simulink model "lab2Sim"  (R2024b)
settings: Solver=VariableStepAuto  StartTime=0.0  StopTime=10.0  MaxStep=5  RelTol=1e-3
values from neighbouring files (symbols this model uses):
  cpp = 1000    [ident.m]    (also in lab2.m)
  Cvs = (cps * ros * Vs)    (= 9240000)    [ident.m]    (also in lab2.m = 92400)
  Cvw = (cpp * rop * Vw)    (= 150000)    [ident.m]    (also in lab2.m)
  czas_skok = 20000    [ident.m]    (also in lab2.m = 10000)
  dFp = 0    [ident.m]    (also in lab2.m)
  dPg = 0.1 * Pg0    (= 800)    [ident.m]    (also in lab2.m = 0)
  dTzew = 0    [ident.m]    (also in lab2.m = 1)
  Fp0 = FpN * 1.0    (= 0.0694444444444)    [ident.m]    (also in lab2.m = 0)
  Ks = Px/(TsN - TzewN)    (= 133.333333333)    [ident.m]    (also in lab2.m)
  Kw = Px/(TwewN - TsN)    (= 933.333333333)    [ident.m]    (also in lab2.m)
  Pg0 = PgN * 1.0    (= 8000)    [ident.m]    (also in lab2.m)
  rop = 1.2    [ident.m]    (also in lab2.m)
  Ts0 = (Kw*Twew0 + Ks*Tzew0) / (Kw + Ks)    (= 15)    [ident.m]    (also in lab2.m = 40)
  Twew0 = (Pg0 + Tzew0*(cpp*rop*Fp0 + ((Ks*Kw)/(Kw + Ks)))) / (cpp*rop*Fp0 + ((Kw * Ks)/(Kw + Ks)))    (= 20)    [ident.m]    (also in lab2.m = 48.5714285714)
  Tzew0 = TzewN    (= -20)    [ident.m]    (also in lab2.m)
settings Model: Creator=Michal  LastModifiedBy=Michal
settings DataIOCC: ReturnWorkspaceOutputs=off

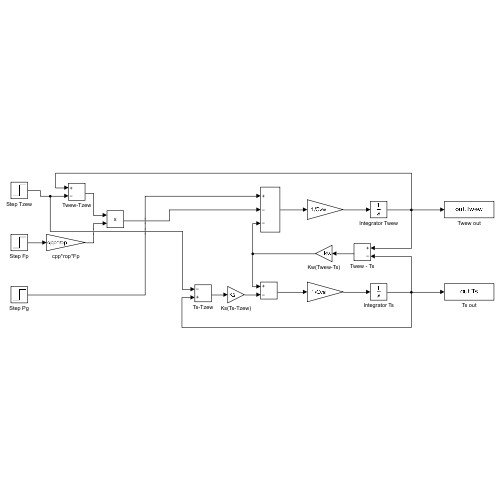
[thumbnail: Simulink's stored preview of the top-level diagram]
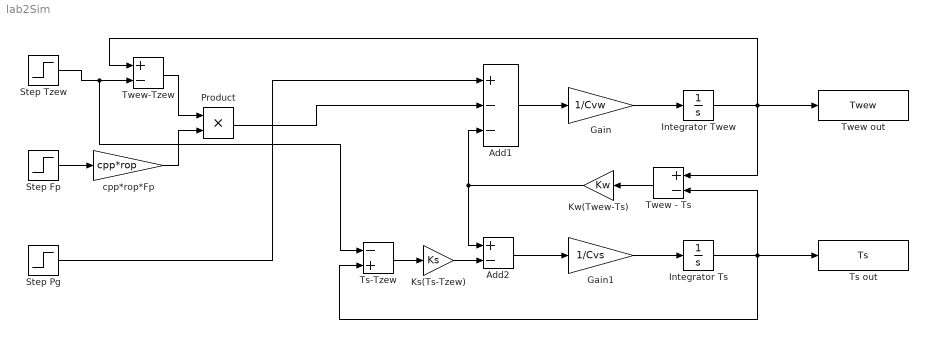
== system lab2Sim ==
  Add1 : Sum  Inputs=+--
  Add2 : Sum  Inputs=+-
  Gain : Gain  Gain=1/Cvw
  Gain1 : Gain  Gain=1/Cvs
  Integrator Ts : Integrator  InitialCondition=Ts0
  Integrator Twew : Integrator  InitialCondition=Twew0
  Ks(Ts-Tzew) : Gain  Gain=Ks
  Kw(Twew-Ts) : Gain  Gain=Kw
  Product : Product
  Step Fp : Step  Time=czas_skok  Before=Fp0  After=Fp0+dFp  SampleTime=0
  Step Pg : Step  Time=czas_skok  Before=Pg0  After=Pg0+dPg  SampleTime=0
  Step Tzew : Step  Time=czas_skok  Before=Tzew0  After=Tzew0+dTzew  SampleTime=0
  Ts out : ToWorkspace  VariableName=Ts  SampleTime=-1
  Ts-Tzew : Sum  Inputs=-+
  Twew - Ts : Sum  Inputs=+-
  Twew out : ToWorkspace  VariableName=Twew  SampleTime=-1
  Twew-Tzew : Sum  Inputs=+-
  cpp*rop*Fp : Gain  Gain=cpp*rop
  wires:
  Integrator Twew/1 -> Twew out/1, Twew-Tzew/1, Twew - Ts/1
  Integrator Ts/1 -> Ts out/1, Twew - Ts/2, Ts-Tzew/2
  Gain/1 -> Integrator Twew/1
  Gain1/1 -> Integrator Ts/1
  Add1/1 -> Gain/1
  Add2/1 -> Gain1/1
  Twew - Ts/1 -> Kw(Twew-Ts)/1
  Step Pg/1 -> Add1/1
  Kw(Twew-Ts)/1 -> Add2/1, Add1/3
  Step Tzew/1 -> Ts-Tzew/1, Twew-Tzew/2
  Step Fp/1 -> cpp*rop*Fp/1
  Twew-Tzew/1 -> Product/1
  cpp*rop*Fp/1 -> Product/2
  Product/1 -> Add1/2
  Ts-Tzew/1 -> Ks(Ts-Tzew)/1
  Ks(Ts-Tzew)/1 -> Add2/2
